simulink library "SampleTime"  (R2019b)
settings: Solver=VariableStepAuto  StartTime=0.0  StopTime=10.0  RelTol=1e-3
settings Model: Creator=Nick  LastModifiedBy=Nick
settings DataIOCC: ReturnWorkspaceOutputs=off
settings DebuggingCC: ArithmeticOperatorsInVariantConditions=warning
settings SFSimCC: CustomCodeUndefinedFunction=UseInterfaceOnly

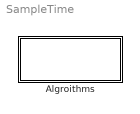
== system SampleTime ==
  Algroithms : Subsystem

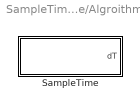
== system SampleTime/Algroithms ==
  SampleTime : Subsystem
      mask Display:
      | color('blue');
      | disp(sprintf(['SampleTime']));

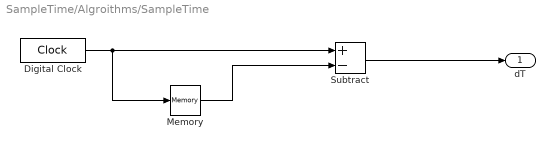
== system SampleTime/Algroithms/SampleTime ==
  Digital Clock : DigitalClock  SampleTime=-1
  Memory : Memory  InheritSampleTime=on
  Subtract : Sum  Inputs=+-
  dT : Outport
  wires:
  Memory/1 -> Subtract/2
  Subtract/1 -> dT/1
  Digital Clock/1 -> Memory/1, Subtract/1
